simulink model "max_rate_test"  (R2018b)
settings: Solver=VariableStepAuto  StartTime=0.0  StopTime=100  RelTol=1e-3
undefined symbols (not defined in the file): fswParams, simParams
libraries: sharedtransform x2, simulink x1, PD_Controller_Lib x1, quat_kinematics_lib x1, sharedutil x1, quat_rectify_lib x1, reaction_wheel_assembly_lib x1, rigid_body_dynamics_lib x1, rwa_allocation_lib x1, sunSeek_lib x1, command_converter_lib x1, two_norm x1
settings Model: Creator=Nick's PC  LastModifiedBy=Nick's PC

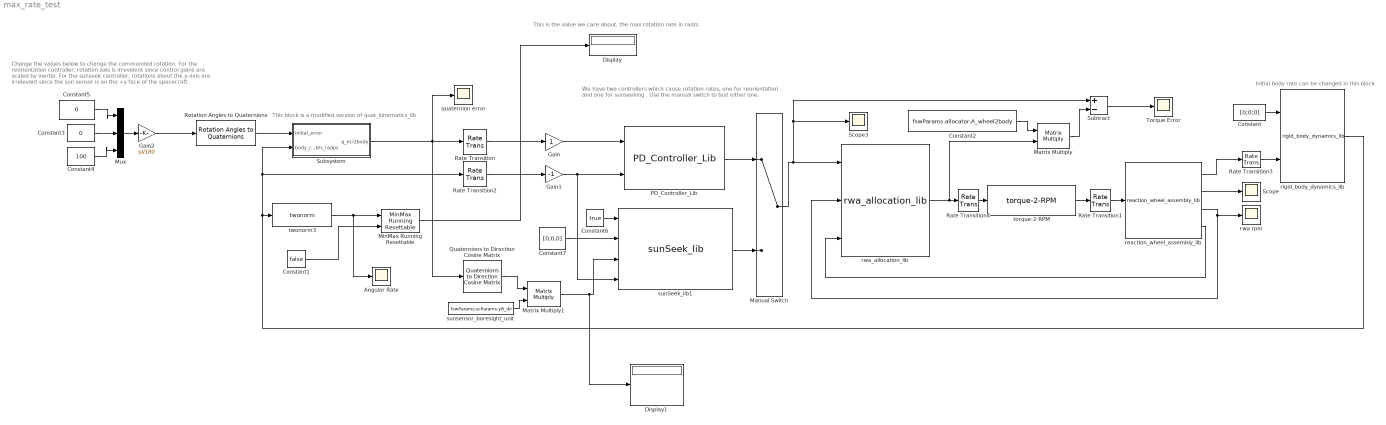
== system max_rate_test ==
  note: We have two controllers which cause rotation rates, one for reorientation and one for sunseeking . Use the manual switch to test either one.
  note: This is the value we care about, the max rotation rate in rad/s.
  note: Change the values below to change the commanded rotation. For the reorientation controller, rotation axis is irrevelent since control gains are scaled by inertia. For the sunseek controller, rotations about the y-axis are irrelevant since the sun sensor is on the +y face of the spacecraft.
  note: Initial body rate can be changed in this block
  note: This block is a modified version of quat_kinematics_lib
  Angular Rate : Scope
  Constant : Constant  Value=[0;0;0]
  Constant1 : Constant  Value=false
  Constant2 : Constant  Value=fswParams.allocator.A_wheel2body
  Constant3 : Constant  Value=0
  Constant4 : Constant  Value=100
  Constant5 : Constant  Value=0
  Constant6 : Constant  Value=true
  Constant7 : Constant  Value=[0,0,0]
  Display : Display
  Display1 : Display
  Gain : Gain
  Gain1 : Gain  Gain=-1
  Gain2 : Gain  Gain=pi/180
  Manual Switch : ManualSwitch
  Matrix Multiply : Product  Multiplication=Matrix(*)
  Matrix Multiply1 : Product  Multiplication=Matrix(*)
  MinMax Running Resettable : simulink/Math Operations/MinMax Running Resettable  Function=max  vinit=0.0
  Mux : Mux  Inputs=3
  PD_Controller_Lib : PD_Controller_Lib/PD_Controller_Lib  SystemSampleTime=-1
  Quaternions to Direction Cosine Matrix : sharedtransform/Quaternions to  Direction Cosine Matrix  aMode=aMode
      settings: SourceProductName=Aerospace Blockset  SourceProductBaseCode=AE
  Rate Transition : RateTransition  OutPortSampleTime=fswParams.sample_time_s
  Rate Transition1 : RateTransition  OutPortSampleTime=simParams.actuators.sample_time_s
  Rate Transition2 : RateTransition  OutPortSampleTime=fswParams.sample_time_s
  Rate Transition3 : RateTransition  OutPortSampleTime=simParams.sample_time_s
  Rate Transition4 : RateTransition  OutPortSampleTime=simParams.actuators.sample_time_s
  Rotation Angles to Quaternions : sharedtransform/Rotation Angles to Quaternions  rotationOrder=ZYX  aMode=aMode
      settings: SourceProductName=Aerospace Blockset  SourceProductBaseCode=AE
  Scope : Scope
  Scope3 : Scope
  Subsystem : Subsystem
  Subtract : Sum  Inputs=+-
  Torque Error : Scope
  quaternion error : Scope
  reaction_wheel_assembly_lib : reaction_wheel_assembly_lib/reaction_wheel_assembly_lib  SystemSampleTime=-1
  rigid_body_dynamics_lib : rigid_body_dynamics_lib/rigid_body_dynamics_lib  SystemSampleTime=-1
  rwa rpm : Scope
  rwa_allocation_lib : rwa_allocation_lib/rwa_allocation_lib  SystemSampleTime=-1
  sunSeek_lib1 : sunSeek_lib/sunSeek_lib  SystemSampleTime=-1
  sunsensor_boresight_unit : Constant  Value=fswParams.scParams.yB_dir
  torque-2-RPM : command_converter_lib/command_converter_lib/torque-2-RPM  SystemSampleTime=-1
      link override Discrete-Time Integrator: InitialCondition=simParams.initialConditions.rwa.h_wheel_Nms
  twonorm3 : two_norm/twonorm  SystemSampleTime=-1
  wires:
  reaction_wheel_assembly_lib/3 -> rwa_allocation_lib/2, rwa rpm/1
  reaction_wheel_assembly_lib/4 -> rwa_allocation_lib/3
  reaction_wheel_assembly_lib/2 -> Scope/1
  Constant/1 -> rigid_body_dynamics_lib/1
  torque-2-RPM/1 -> Rate Transition1/1
  Rate Transition1/1 -> reaction_wheel_assembly_lib/1
  reaction_wheel_assembly_lib/1 -> Rate Transition3/1
  Rate Transition3/1 -> rigid_body_dynamics_lib/2
  rigid_body_dynamics_lib/1 -> twonorm3/1, Rate Transition2/1, Subsystem/2(body_rates_radps)
  Subsystem/1(q_eci2body) -> quaternion error/1, Quaternions to Direction Cosine Matrix/1, Rate Transition/1
  rwa_allocation_lib/1 -> Rate Transition4/1, Matrix Multiply/2
  Rate Transition/1 -> Gain/1
  Gain/1 -> PD_Controller_Lib/1
  Rate Transition2/1 -> Gain1/1
  twonorm3/1 -> MinMax Running Resettable/1, Angular Rate/1
  Subtract/1 -> Torque Error/1
  Matrix Multiply/1 -> Subtract/2
  Constant2/1 -> Matrix Multiply/1
  Rate Transition4/1 -> torque-2-RPM/1
  PD_Controller_Lib/1 -> Manual Switch/1
  Gain1/1 -> sunSeek_lib1/4, PD_Controller_Lib/2
  Manual Switch/1 -> Subtract/1, Scope3/1, rwa_allocation_lib/1
  Rotation Angles to Quaternions/1 -> Subsystem/1(initial_error)
  Gain2/1 -> Rotation Angles to Quaternions/1
  Constant3/1 -> Mux/2
  Mux/1 -> Gain2/1
  Constant4/1 -> Mux/3
  Constant5/1 -> Mux/1
  MinMax Running Resettable/1 -> Display/1
  Constant1/1 -> MinMax Running Resettable/2
  sunSeek_lib1/1 -> Manual Switch/2
  Constant6/1 -> sunSeek_lib1/1
  Constant7/1 -> sunSeek_lib1/2
  sunsensor_boresight_unit/1 -> Matrix Multiply1/2
  Matrix Multiply1/1 -> Display1/1, sunSeek_lib1/3
  Quaternions to Direction Cosine Matrix/1 -> Matrix Multiply1/1

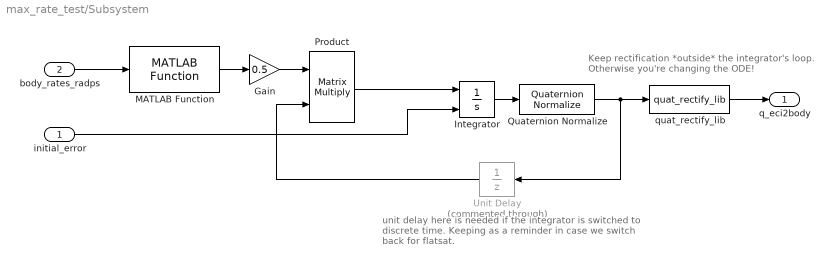
== system max_rate_test/Subsystem ==
  note: unit delay here is needed if the integrator is
      | switched to discrete time. Keeping as a reminder
      | in case we switch back for flatsat.
  note: Keep rectification *outside* the integrator's
      | loop. Otherwise you're changing the ODE!
  initial_error : Inport
  body_rates_radps : Inport  Port=2
  Gain : Gain  Gain=0.5
  Integrator : Integrator  InitialConditionSource=external  InitialCondition=simParams.initialConditions.q_eci2body
  MATLAB Function : quat_kinematics_lib/quat_kinematics_lib/MATLAB Function  SystemSampleTime=-1
  Product : Product  Multiplication=Matrix(*)
  Quaternion Normalize : sharedutil/Quaternion Normalize  aMode=aMode
      settings: SourceProductName=Aerospace Blockset  SourceProductBaseCode=AE
  Unit Delay : UnitDelay  Commented=through  InitialCondition=simParams.initialConditions.q_eci2body  SampleTime=-1
  quat_rectify_lib : quat_rectify_lib/quat_rectify_lib
  q_eci2body : Outport
  wires:
  MATLAB Function/1 -> Gain/1
  Gain/1 -> Product/1
  Integrator/1 -> Quaternion Normalize/1
  quat_rectify_lib/1 -> q_eci2body/1
  Product/1 -> Integrator/1
  Unit Delay/1 -> Product/2
  Quaternion Normalize/1 -> quat_rectify_lib/1, Unit Delay/1
  body_rates_radps/1 -> MATLAB Function/1
  initial_error/1 -> Integrator/2
